simulink model "PlaneSimulationModel_withSensors_r17"  (R2022b)
settings: Solver=FixedStepAuto  StartTime=0.0  StopTime=20  FixedStep=0.0025  RelTol=1e-3
libraries: simulink x12
(part 2 of 2)

== matlab function PlaneSimulationModel_withSensors_r17/NAVIGATION SENSOR MODEL/GPS Simulator ==
  data: base_lat input int32; base_lng input int32; sigma parameter; NewDataGPS output; base_alt input single; sat_out output; fix_out output; x input; lat_out output int32; y input; z input; sat input uint8; error_type input uint8; lng_out output int32; dt parameter single; gps_delay parameter single; f_gps parameter single; alt_out output single; sigma_alt parameter; vx_out output; vy_out output; vz_out output; hAcc output; vAcc output; sAcc output
function [NewDataGPS, sat_out,fix_out,lat_out,lng_out,alt_out,vx_out,vy_out,vz_out, hAcc, vAcc, sAcc] = fcn(base_lat, base_lng, sigma,base_alt,x,y,z,sat,error_type, dt, gps_delay, f_gps,  sigma_alt)
persistent zoh; if isempty(zoh) zoh=single(0);end
persistent init; if isempty(init) init=false;end
persistent lat; if isempty(lat) lat=int32(0);end
persistent lng; if isempty(lng) lng=int32(0);end
persistent alt; if isempty(alt) alt=single(0);end
persistent vx_delay; if isempty(vx_delay) vx_delay=single(0);end
persistent vy_delay; if isempty(vy_delay) vy_delay=single(0);end
persistent vz_delay; if isempty(vz_delay) vz_delay=single(0);end
persistent ile_probek_delay; if isempty(ile_probek_delay) ile_probek_delay=single(0);end
persistent ile_probek_zoh; if isempty(ile_probek_zoh) ile_probek_zoh=single(0);end
persistent i; if isempty(i) i=single(0);end
persistent x_out; if isempty(x_out) x_out=single(0);end
persistent buff; if isempty(buff) buff=single(zeros(5,3));end
persistent rx_srednia; if isempty(rx_srednia) rx_srednia=single(0);end
persistent ry_srednia; if isempty(ry_srednia) ry_srednia=single(0);end
persistent rz_srednia; if isempty(rz_srednia) rz_srednia=single(0);end
persistent licznik1; if isempty(licznik1) licznik1=single(0);end
persistent licznik2; if isempty(licznik2) licznik2=single(0);end
persistent licznik3; if isempty(licznik3) licznik3=single(0);end
persistent x_delay_old; if isempty(x_delay_old) x_delay_old=single(0);end
persistent y_delay_old; if isempty(y_delay_old) y_delay_old=single(0);end
persistent z_delay_old; if isempty(z_delay_old) z_delay_old=single(0);end

persistent lat_plus_old; if isempty(lat_plus_old) lat_plus_old=false;end
persistent lng_plus_old; if isempty(lng_plus_old) lng_plus_old=false;end

persistent timeStart; if isempty(timeStart) timeStart=single(0);end


if(~init) 
    init=true;
    ile_probek_zoh = 1/single(f_gps)/single(dt);
    ile_probek_delay = single(gps_delay)*0.001/(1/single(f_gps))+1;
end


NewDataGPS = uint8(0);


xmin=-0.4;
xmax=0.4;
n=single(500);
t_sin=rand(1,1,'single')*(xmax-xmin)+xmin;
licznik1 = licznik1 + t_sin;
if(licznik1>=360)
    licznik1 = single(0);
end

if(error_type==1)
    sat = uint8(3);
elseif(error_type==2)
    sat = uint8(0);
end

if(timeStart <= 5)
    if(timeStart <= 1 && sat > 0)
        sat = uint8(0);
    elseif(timeStart <= 1.5 && sat > 1)
        sat = uint8(1);
    elseif(timeStart <= 2 && sat > 2)
        sat = uint8(2);
    elseif(timeStart <= 2.2 && sat > 3)
        sat = uint8(3);
    end
    timeStart = timeStart + single(dt);
end


if(error_type>=3)
    k = single(error_type);
else
    k = skalowanie(0,18,1.5,0.5,single(sat));
end


rx = sind(licznik1)*sigma*k+rand(1,1,'single')/4*k;
rx_srednia=rx_srednia*n;
rx_srednia=rx_srednia+rx;
rx_srednia=rx_srednia/(n+1);


t_sin=rand(1,1,'single')*(xmax-xmin)+xmin;
licznik2 = licznik2 + t_sin;
if(licznik2>=360)
    licznik2 = single(0);
end
ry = sind(licznik1)*sigma*k+rand(1,1,'single')/4*k;
ry_srednia=ry_srednia*n;
ry_srednia=ry_srednia+ry;
ry_srednia=ry_srednia/(n+1);


t_sin=rand(1,1,'single')*(xmax-xmin)+xmin;
licznik3 = licznik3 + t_sin;
if(licznik3>=360)
    licznik3 = single(0);
end
rz = sind(licznik1)*sigma_alt*k+rand(1,1,'single')/4*k;
rz_srednia=rz_srednia*n;
rz_srednia=rz_srednia+rz;
rz_srednia=rz_srednia/(n+1);

if(zoh>ile_probek_zoh-1)
    i=i+1;
    if(i>ile_probek_delay)
        i=single(1);
    end
    
    buff(i,1)=x;
    buff(i,2)=y;
    buff(i,3)=z;

    zoh=single(0);
    if(i+1>ile_probek_delay)
        x_delay=buff(1,1);
        y_delay=buff(1,2);
        z_delay=buff(1,3);
    else
        x_delay=buff(i+1,1);
        y_delay=buff(i+1,2);
        z_delay=buff(i+1,3);
    end
    
    x_delay = x_delay + rx_srednia;
    y_delay = y_delay + ry_srednia;
    z_delay = z_delay + rz_srednia;

    if(error_type~=2)
        % error type 2 == NO DATA
        NewDataGPS = uint8(1);
        [lat_d, lng_d] = get_NE_from_vector(base_lat, base_lng, [x_delay y_delay]);
        lat  = int32(lat_d);
        lng  = int32(lng_d);

        if(base_alt >=0)
            alt = base_alt + z_delay;
        else
            alt = base_alt + z_delay;
        end
        vx_delay = (x_delay - x_delay_old)/(1/f_gps);
        vy_delay = (y_delay - y_delay_old)/(1/f_gps);
        vz_delay = (z_delay - z_delay_old)/(1/f_gps);
    end
    x_delay_old = x_delay;
    y_delay_old = y_delay;
    z_delay_old = z_delay;

end
zoh=zoh+1;

sat_out = uint8(sat);
switch sat
    case {0,1,2}
        fix = uint8(0);
        hAcc = single(99);
        vAcc = single(99);
        sAcc = single(99);
    case 3
        fix = uint8(2);
        hAcc = single(sigma*10);
        vAcc = single(sigma_alt*10);
        sAcc = single(sigma_alt*10);
    otherwise
        fix = uint8(3);
        hAcc = single(sigma);
        vAcc = single(sigma_alt);
        sAcc = single(sigma_alt);
end
fix_out = fix;
if(fix)
    lat_out = lat;
    lng_out = lng;
    alt_out = alt;
    vx_out = vx_delay;
    vy_out = vy_delay;
    vz_out = vz_delay;
else
    lat_out = int32(0);
    lng_out = int32(0);
    alt_out = single(0);
    vx_out = single(0);
    vy_out = single(0);
    vz_out = single(0);
end

end



function [lat_dest_pos, lon_dest_pos]  = get_NE_from_vector(base_lat, base_lon, vect_xy)

    LATLON_TO_M  = double(0.01113195);
    scale = double(cos((double(base_lat) * 1.0e-7 * pi/180)));
    y_offs = double(ograniczenie(single(scale),0.1, 1));

    lat_dest_pos_d = double((vect_xy(1,1)/LATLON_TO_M));
    lon_dest_pos_d = double((vect_xy(1,2)/(y_offs * LATLON_TO_M)));
    
    lat_dest_pos = int32(lat_dest_pos_d) + base_lat;
    lon_dest_pos = int32(lon_dest_pos_d) + base_lon;
end
